simulink model "Wind_PMSG_Rectifier"  (Simulink 7.1)
settings: Solver=ode23tb  StartTime=0.0  StopTime=10.0  RelTol=1e-3
undefined symbols (not defined in the file or in its folder): c1, c2, c3, c4, c5, c6, DiscIntNeverNeededParam
libraries: powerlib x20, powerlib_extras x10, simulink x1
settings Model: Creator=jagan  LastModifiedBy=jagan

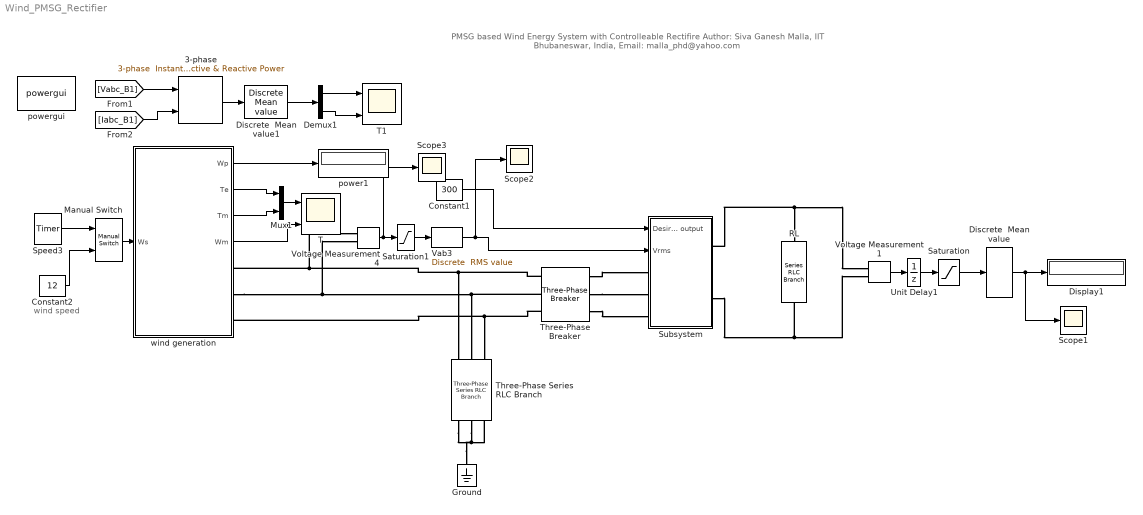
== system Wind_PMSG_Rectifier ==
  note: wind speed
  note: PMSG based Wind Energy System with Controlleable Rectifire
      | Author: Siva Ganesh Malla, IIT Bhubaneswar, India, Email: malla_phd@yahoo.com
  "3-phase " : powerlib_extras/Measurements/3-phase  Instantaneous  Active & Reactive Power  DialogController=POWERSYS.PowerSysDialog  SystemSampleTime=-1
  Constant1 : Constant  Value=300  OutDataType=sfix(16)  OutScaling=2^0
  Constant2 : Constant  Value=12  OutDataType=sfix(16)  OutScaling=2^0
  Demux1 : Demux  Outputs=2
  Discrete  Mean value : powerlib_extras/Discrete Measurements/Discrete  Mean value  DialogController=POWERSYS.PowerSysDialog  SystemSampleTime=-1  Freq=50*6  Vinit=0  Ts=50e-6
  Discrete  Mean value1 : powerlib_extras/Discrete Measurements/Discrete  Mean value  DialogController=POWERSYS.PowerSysDialog  SystemSampleTime=-1  Freq=50  Vinit=0  Ts=20e-6
  Display1 : Display
  Ground : powerlib/Elements/Ground  Orientation=down  DialogController=POWERSYS.PowerSysDialog  PhysicalDomain=powersysdomain  SubClassName=unknown  LeftPortType=p1  RightPortType=p1  LConnTagsString=a
  Manual Switch : simulink/Signal Routing/Manual Switch  SystemSampleTime=-1  sw=0  action=0  varsize=off
  Mux1 : Mux  Inputs=2
  RL : powerlib/Elements/Series RLC Branch  Orientation=down  DialogController=POWERSYS.PowerSysDialog  PhysicalDomain=powersysdomain  SubClassName=unknown  LeftPortType=p1  RightPortType=p1  LConnTagsString=__new0  RConnTagsString=__new0  BranchType=RL  Resistance=10  Inductance=50e-3  SetiL0=off  InitialCurrent=0  Capacitance=1e-6  Setx0=off  InitialVoltage=0  Measurements=None
  Saturation : Saturate  UpperLimit=1000  LowerLimit=-1000  OutDataType=sfix(16)  OutScaling=2^0
  Saturation1 : Saturate  UpperLimit=1000  LowerLimit=-1000  OutDataType=sfix(16)  OutScaling=2^0
  Scope1 : Scope
      settings: TimeRange=0.02  YMin=270  YMax=355  SaveName=ScopeData3
  Scope2 : Scope
      settings: TimeRange=0.02  YMin=423  YMax=438  SaveName=ScopeData5
  Scope3 : Scope
      settings: TimeRange=0.02  YMin=-1000  YMax=700  SaveName=ScopeData6
  Speed3 : powerlib_extras/Control  Blocks/Timer  DialogController=POWERSYS.PowerSysDialog  SystemSampleTime=-1  t=[0 3 5]  e=[12 7 12]
  Subsystem : Subsystem
  T : Scope  NumInputPorts=2
      settings: YMin=39.75~152.46  YMax=39.97~152.59  SaveName=Wind_MPPT  SampleInput=on  SampleTime=100e-6
  T1 : Scope  NumInputPorts=2
      settings: YMin=4380~-4e-014  YMax=4520~3.5e-014  SaveName=Wind_MPPT1  SampleInput=on  SampleTime=100e-6
  Three-Phase Series RLC Branch : powerlib/Elements/Three-Phase Series RLC Branch  Orientation=down  DialogController=POWERSYS.PowerSysDialog  PhysicalDomain=powersysdomain  SubClassName=unknown  LeftPortType=p1  RightPortType=p1  LConnTagsString=A|B|C  RConnTagsString=A|B|C  BranchType=R  Resistance=800  Inductance=1e-3  Capacitance=1e-6  Measurements=None
  Three-Phase Breaker : powerlib/Elements/Three-Phase Breaker  DialogController=POWERSYS.PowerSysDialog  SystemSampleTime=-1  InitialState=open  SwitchA=on  SwitchB=on  SwitchC=on  SwitchTimes=[1 10]  External=off  BreakerResistance=0.001  SnubberResistance=1e6  SnubberCapacitance=inf  Measurements=None
  Unit Delay1 : UnitDelay  SampleTime=-1
  Vab3 : powerlib_extras/Discrete Measurements/Discrete  RMS value  DialogController=POWERSYS.PowerSysDialog  SystemSampleTime=-1  Freq=50  Mag_Init=0  Ts=20e-6
  Voltage Measurement1 : powerlib/Measurements/Voltage Measurement  DialogController=POWERSYS.PowerSysDialog  SystemSampleTime=-1  PhasorSimulation=off  OutputType=Complex  PSBequivalent=0
  Voltage Measurement4 : powerlib/Measurements/Voltage Measurement  DialogController=POWERSYS.PowerSysDialog  SystemSampleTime=-1  PhasorSimulation=off  OutputType=Complex  PSBequivalent=0
  power1 : Display
      settings: SampleTime=1e-3
  powergui : powerlib/powergui  SystemSampleTime=-1  SimulationMode=Discrete  SampleTime=20e-6  frequency=60  SPID=off  SwTol=0  Interpol=off  x0status=blocks  echomessages=off  HookPort=off  FunctionMessages=off  EnableUseOfTLC=off  RestoreLinks=warning  frequencyindice=0  Frange=[0:2:500]  Ylog=off  Xlog=on  ShowGrid=off  save=off  variable=ZData  ZoomFFT=on  StartTime=0.0  cycles=1  DisplayStyle=1  fundamental=60  FreqAxis=off  MaxFrequency=1000  frequencyindicesteady=1  RmsSteady=1  display=off  Ts=0  methode=off
  wind generation : Subsystem
  wires:
  [Vabc_B1] -> "3-phase "/1
  [Iabc_B1] -> "3-phase "/2
  "3-phase "/1 -> Discrete  Mean value1/1
  Discrete  Mean value1/1 -> Demux1/1
  Demux1/1 -> T1/1
  Speed3/1 -> Manual Switch/1
  Constant2/1 -> Manual Switch/2
  Manual Switch/1 -> wind generation/1(Ws)
  Mux1/1 -> T/1
  wind generation/1(Wp) -> power1/1
  wind generation/2(Te) -> Mux1/1
  wind generation/3(Tm) -> Mux1/2
  wind generation/4(Wm) -> T/2
  Demux1/2 -> T1/2
  Voltage Measurement4/1 -> Saturation1/1, Scope3/1
  Saturation1/1 -> Vab3/1
  Vab3/1 -> Subsystem/2(Vrms), Scope2/1
  Constant1/1 -> Subsystem/1(Desird output)
  Discrete  Mean value/1 -> Display1/1, Scope1/1
  Voltage Measurement1/1 -> Unit Delay1/1
  Saturation/1 -> Discrete  Mean value/1
  Unit Delay1/1 -> Saturation/1
  connections:
  wind generation/RConn2 -- Voltage Measurement4/LConn2 -- Three-Phase Breaker/LConn2 -- Three-Phase Series RLC Branch/LConn2
  Three-Phase Breaker/RConn1 -- Subsystem/LConn1
  Three-Phase Breaker/RConn3 -- Subsystem/LConn3
  Subsystem/RConn1 -- Voltage Measurement1/LConn1 -- RL/LConn1
  Subsystem/RConn2 -- Voltage Measurement1/LConn2 -- RL/RConn1
  wind generation/RConn3 -- Three-Phase Breaker/LConn3 -- Three-Phase Series RLC Branch/LConn3
  Three-Phase Breaker/RConn2 -- Subsystem/LConn2
  Three-Phase Breaker/LConn1 -- Three-Phase Series RLC Branch/LConn1 -- wind generation/RConn1 -- Voltage Measurement4/LConn1
  Ground/LConn1 -- Three-Phase Series RLC Branch/RConn1 -- Three-Phase Series RLC Branch/RConn3 -- Three-Phase Series RLC Branch/RConn2

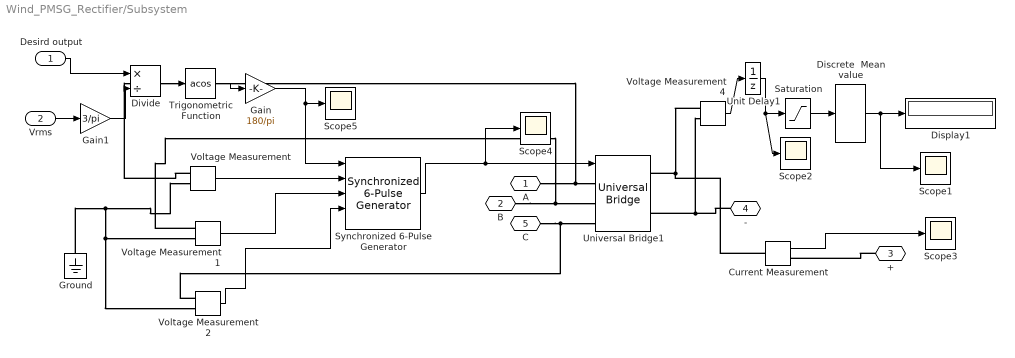
== system Wind_PMSG_Rectifier/Subsystem ==
  Desird output : Inport
  Vrms : Inport  Port=2
  Current Measurement : powerlib/Measurements/Current Measurement  DialogController=POWERSYS.PowerSysDialog  SystemSampleTime=-1  PhasorSimulation=off  OutputType=Complex  PSBequivalent=0
  Discrete  Mean value : powerlib_extras/Discrete Measurements/Discrete  Mean value  DialogController=POWERSYS.PowerSysDialog  SystemSampleTime=-1  Freq=50*6  Vinit=0  Ts=50e-6
  Display1 : Display
  Divide : Product  Inputs=*/  OutDataType=sfix(16)  OutScaling=2^-10
  Gain : Gain  Gain=180/pi  ParameterDataType=sfix(16)  ParameterScaling=2^0  OutDataType=sfix(16)  OutScaling=2^0
  Gain1 : Gain  Gain=3/pi  ParameterDataType=sfix(16)  ParameterScaling=2^0  OutDataType=sfix(16)  OutScaling=2^0
  Ground : powerlib/Elements/Ground  Orientation=down  DialogController=POWERSYS.PowerSysDialog  PhysicalDomain=powersysdomain  SubClassName=unknown  LeftPortType=p1  RightPortType=p1  LConnTagsString=a
  Saturation : Saturate  UpperLimit=1000  LowerLimit=-1000  OutDataType=sfix(16)  OutScaling=2^0
  Scope{1..5} (5 alike) : Scope
      Scope1 settings: TimeRange=0.02  YMin=-25  YMax=325
      Scope2 settings: TimeRange=0.02  YMin=-250  YMax=550
      Scope3 settings: TimeRange=0.02  YMin=25.75  YMax=28.5  SaveName=ScopeData2
      Scope4 settings: TimeRange=0.02  YMin=0  YMax=1  SaveName=ScopeData4
      Scope5 settings: TimeRange=0.02  YMin=-1  YMax=1  SaveName=ScopeData7
  Synchronized 6-Pulse Generator : powerlib_extras/Control  Blocks/Synchronized 6-Pulse Generator  DialogController=POWERSYS.PowerSysDialog  SystemSampleTime=-1  freq=25  pwidth=50  Double_Pulse=off
  Trigonometric Function : Trigonometry  Operator=acos
  Unit Delay1 : UnitDelay  SampleTime=-1
  Universal Bridge1 : powerlib/Power Electronics/Universal Bridge  DialogController=POWERSYS.PowerSysDialog  SystemSampleTime=-1  Arms=3  SnubberResistance=1e5  SnubberCapacitance=inf  Device=Thyristors  Ron=1e-3  Lon=0  ForwardVoltages="[  0  0  ]"  ForwardVoltage=0  GTOparameters=[ 10e-6 , 20e-6 ]  IGBTparameters=[ 1e-6 , 2e-6 ]  Measurements=None  converterType=Rectifier
  Voltage Measurement{,1..2,4} (4 alike) : powerlib/Measurements/Voltage Measurement  DialogController=POWERSYS.PowerSysDialog  SystemSampleTime=-1  PhasorSimulation=off  OutputType=Complex  PSBequivalent=0
  A : PMIOPort  Port=1  Side=Left
  B : PMIOPort  Port=2  Side=Left
  + : PMIOPort  Orientation=left  Port=3  Side=Right
  - : PMIOPort  Orientation=left  Port=4  Side=Right
  C : PMIOPort  Port=5  Side=Left
  wires:
  Voltage Measurement/1 -> Synchronized 6-Pulse Generator/2
  Voltage Measurement1/1 -> Synchronized 6-Pulse Generator/3
  Voltage Measurement2/1 -> Synchronized 6-Pulse Generator/4
  Synchronized 6-Pulse Generator/1 -> Universal Bridge1/1, Scope4/1
  Voltage Measurement4/1 -> Unit Delay1/1
  Current Measurement/1 -> Scope3/1
  Divide/1 -> Trigonometric Function/1
  Trigonometric Function/1 -> Gain/1
  Gain/1 -> Synchronized 6-Pulse Generator/1, Scope5/1
  Discrete  Mean value/1 -> Display1/1, Scope1/1
  Desird output/1 -> Divide/1
  ? -> Synchronized 6-Pulse Generator/5
  Gain1/1 -> Divide/2
  Vrms/1 -> Gain1/1
  Saturation/1 -> Discrete  Mean value/1
  Unit Delay1/1 -> Scope2/1, Saturation/1
  connections:
  Current Measurement/LConn1 -- Voltage Measurement4/LConn1 -- Universal Bridge1/RConn1
  A/RConn1 -- Universal Bridge1/LConn1 -- Voltage Measurement/LConn1
  -/RConn1 -- Universal Bridge1/RConn2 -- Voltage Measurement4/LConn2
  Voltage Measurement2/LConn1 -- C/RConn1 -- Universal Bridge1/LConn3
  +/RConn1 -- Current Measurement/RConn1
  Voltage Measurement1/LConn1 -- B/RConn1 -- Universal Bridge1/LConn2
  Voltage Measurement/LConn2 -- Ground/LConn1 -- Voltage Measurement2/LConn2 -- Voltage Measurement1/LConn2

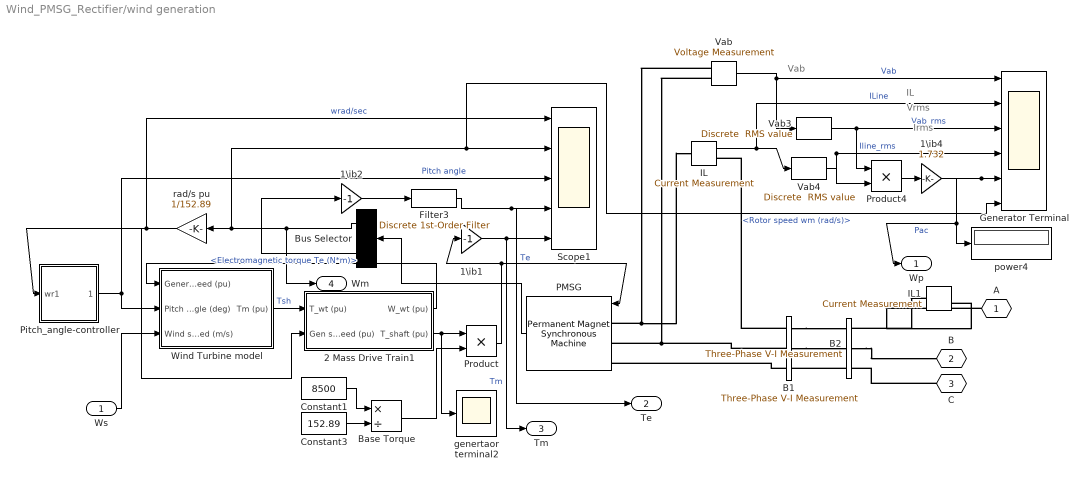
== system Wind_PMSG_Rectifier/wind generation ==
  note: Vab
  note: IL
  note: Vrms
  note: Irms
  Ws : Inport  OutDataType=sfix(16)  OutScaling=2^0
  1\ib1 : Gain  Gain=-1  ParameterDataType=sfix(16)  ParameterScaling=2^0  OutDataType=sfix(16)  OutScaling=2^0  SaturateOnIntegerOverflow=on  OutDataTypeStr=Inherit: Same as input  ParamDataTypeStr=Inherit: Same as input
  1\ib2 : Gain  Gain=-1  ParameterDataType=sfix(16)  ParameterScaling=2^0  OutDataType=sfix(16)  OutScaling=2^0  SaturateOnIntegerOverflow=on  OutDataTypeStr=Inherit: Same as input  ParamDataTypeStr=Inherit: Same as input
  1\ib4 : Gain  Gain=1.732  ParameterDataType=sfix(16)  ParameterScaling=2^0  OutDataType=sfix(16)  OutScaling=2^0  SaturateOnIntegerOverflow=on  OutDataTypeStr=Inherit: Same as input  ParamDataTypeStr=Inherit: Same as input
  2 Mass Drive Train1 : Subsystem
  B1 : powerlib/Measurements/Three-Phase V-I Measurement  DialogController=POWERSYS.PowerSysDialog  SystemSampleTime=-1  VoltageMeasurement=phase-to-ground  SetLabelV=on  LabelV=Vabc_B1  Vpu=off  CurrentMeasurement=yes  SetLabelI=on  LabelI=Iabc_B1  Ipu=off  Pbase=100e6  Vbase=500e3  OutputType=Magnitude  PhasorSimulation=off  PSBequivalent=0
  "B2 " : powerlib/Measurements/Three-Phase V-I Measurement  DialogController=POWERSYS.PowerSysDialog  SystemSampleTime=-1  VoltageMeasurement=no  SetLabelV=on  LabelV=Vabc_B2  Vpu=off  CurrentMeasurement=no  SetLabelI=on  LabelI=Iabc_B2  Ipu=off  Pbase=100e6  Vbase=500e3  OutputType=Magnitude  PhasorSimulation=off  PSBequivalent=0
  Base Torque : Product  Inputs=*/  OutDataType=sfix(16)  OutScaling=2^0  RndMeth=Zero
  Bus Selector : BusSelector  Orientation=left  OutputSignals=Rotor speed wm (rad/s),Electromagnetic torque Te (N*m)
  Constant1 : Constant  Value=8500  OutDataType=sfix(16)  OutScaling=2^0
  Constant3 : Constant  Value=152.89  OutDataType=sfix(16)  OutScaling=2^0
  Filter3 : powerlib_extras/Discrete  Control Blocks/Discrete 1st-Order Filter  DialogController=POWERSYS.PowerSysDialog  SystemSampleTime=-1  FilterType=Lowpass  Tc=1e-3  Ts=20e-6  Initialize=off  Vac_Init=[0.8 -25 60]  Vdc_Init=-0.4  PlotResponse=off  param1=[1 500 0.1]
  Generator Terminal : Scope  NumInputPorts=6
      settings: YMin=-750~-1~450~0.525~410~175.15  YMax=750~1~477.5~0.56~460~175.4  SaveName=Generator_Terminal  SampleInput=on  SampleTime=100e-6
  IL : powerlib/Measurements/Current Measurement  DialogController=POWERSYS.PowerSysDialog  SystemSampleTime=-1  PhasorSimulation=off  OutputType=Complex  PSBequivalent=0
  IL1 : powerlib/Measurements/Current Measurement  DialogController=POWERSYS.PowerSysDialog  SystemSampleTime=-1  PhasorSimulation=off  OutputType=Complex  PSBequivalent=0
  PMSG : powerlib/Machines/Permanent Magnet Synchronous Machine  Orientation=left  DialogController=POWERSYS.PowerSysDialog  SystemSampleTime=-1  FluxDistribution=Sinusoidal  MechanicalLoad=Torque Tm  PresetModel=No  ShowDetailedParameters=on  Resistance=0.425  Inductance=8.5e-3  dqInductances=[0.0082 0.0082]  MachineConstant=Flux linkage established by magnets (V.s)  Flux=0.433  VoltageCst=392.6876  TorqueCst=3.2475  Flat=120  Mechanical=[0.01197 0.001189 5]  PolePairs=5  InitialConditions=[0,0, 0,0]  TsPowergui=0  TsBlock=-1
  Pitch_angle-controller : Subsystem
  Product : Product  OutDataType=sfix(16)  OutScaling=2^0  RndMeth=Zero
  Product4 : Product  OutDataType=sfix(16)  OutScaling=2^0  RndMeth=Zero
  Scope1 : Scope  NumInputPorts=5
      settings: YMin=0.993~151.8~-1~37.5~40.05  YMax=1~152.8~1~42.5~40.325  SaveName=ScopeData90  SampleInput=on  SampleTime=100e-6
  Vab : powerlib/Measurements/Voltage Measurement  DialogController=POWERSYS.PowerSysDialog  SystemSampleTime=-1  PhasorSimulation=off  OutputType=Complex  PSBequivalent=0
  Vab3 : powerlib_extras/Discrete Measurements/Discrete  RMS value  DialogController=POWERSYS.PowerSysDialog  SystemSampleTime=-1  Freq=50  Mag_Init=0  Ts=20e-6
  Vab4 : powerlib_extras/Discrete Measurements/Discrete  RMS value  DialogController=POWERSYS.PowerSysDialog  SystemSampleTime=-1  Freq=50  Mag_Init=0  Ts=20e-6
  Wind Turbine model : Subsystem  AncestorBlock=DRlib/Wind Generation/Wind Turbine  DialogController=POWERSYS.PowerSysDialog  mask(Wind Turbine){Pnom=8.5e3, Pelec_base=8.5e3/0.9, wind_base=12, P_wind_base=0.8, speed_nom=1, pitch_angle=0, DisplayTurbChar=off, c1_c6=[0.51763          116          0.4            5           21     0.006795], cp_nom=0.48, lambda_nom=8.1}
      mask prompts: Pnom "Nominal mechanical output power (W):"; Pelec_base "Base power of the electrical generator (VA):"; wind_base "Base wind speed (m/s):"; P_wind_base "Maximum power at base wind speed (pu of nominal mechanical power):"; speed_nom "Base rotational speed (p.u. of base generator speed):"; pitch_angle "Pitch angle beta to display wind-turbine power characteristics (beta >=0)  (deg):"; DisplayTurbChar "Display wind turbine power characteristics"
      mask help:
      | This block implements a variable pitch wind turbine model. The performance coefficient Cp of the turbine is the mechanical output power of the turbine divided by wind power and a function of wind speed, rotational speed, and pitch angle (beta). Cp reaches its maximum value at zero beta. Select the wind-turbine power characteristics display to plot the turbine characteristics at the specified pitch angle.
      |
      | The first input is the generator speed in per unit of the generator base speed. For a synchronous or asynchronous generator, the base speed is the synchronous speed. For a permanent-magnet generator, the base speed is defined as the speed producing nominal voltage at  no load. The second input is the blade pitch angle (beta) in degrees. The third input is the wind speed in m/s.
      |
      | The output is the torque applied to the generator shaft in per unit of the generator ratings.
      |
      | The turbine inertia must be added to the generator inertia.
      mask init:
      | %Wind turbine typical characteristic data
      | %c2=116;c3=0.4;c4=5;c5=21;
      | %Computation of c1 and c6 for lambda_nom et cpmax
      | %lambda_nom=8.1;
      | %cp_max=0.48;
      | %cp_nom=cp_max;
      | 
      | %lambda_i_nom=1/(1/lambda_nom-0.035);
      | %k_nom=-(c2*c5/lambda_i_nom-c4*c5-c2)*exp(-c5/lambda_i_nom)/lambda_nom^2;
      | %c1=cp_max/((c2/lambda_i_nom-c4)*exp(-c5/lambda_i_nom)+k_nom*lambda_nom);
      | %c6=k_nom*c1;
      | power_initmask();
      mask Help: web(psbhelp);
      mask CallbackString:
      | ParVisible={'on','on','on','on','on','on','on','off','off','off',};
      | set_param(gcb,'MaskVisibilities',ParVisible);
      | c1_c6=str2num(get_param(gcb,'c1_c6'));
      | c1=c1_c6(1);c2=c1_c6(2);c3=c1_c6(3);c4=c1_c6(4);c5=c1_c6(5);c6=c1_c6(6);||||||DisplayTurbChar=get_param(gcb,'DisplayTurbChar');
      | 
      | if strcmp(DisplayTurbChar,'on')
      |     fig_num=figure;
      | 	clf(fig_num);
      | 	[speed_nom,wind_base,P_wind_base,pitch_angle]=getSPSmaskvalues(gcb,{'speed_nom','wind_base','P_wind_base','pitch_angle'});
      | 	[c1_c6,lambda_nom,cp_nom]=getSPSmaskvalues(gcb,{'c1_c6','lambda_nom','cp_nom'});
      | 	c1=c1_c6(1);c2=c1_c6(2);c3=c1_c6(3);c4=c1_c6(4);c5=c1_c6(5);c6=c1_c6(6);
      | 
      | 	%Wind turbine typical characteristic data
      |     %c2=116;c3=0.4;c4=5;c5=21;
      |     %Computation of c1 and c6 for lambda_nom et cpmax
      |     %lambda_nom=8.1;
      |     %cp_max=0.48;
      |     %cp_nom=cp_max;
      | 
      |     %lambda_i_nom=1/(1/lambda_nom-0.035);
      |     %k_nom=-(c2*c5/lambda_i_nom-c4*c5-c2)*exp(-c5/lambda_i_nom)/lambda_nom^2;
      |     %c1=cp_max/((c2/lambda_i_nom-c4)*exp(-c5/lambda_i_nom)+k_nom*lambda_nom);
      |     %c6=k_nom*c1;
      | 
      | 	wr_elec_pu=1e-3:0.01:1.5;;
      |     wr_mec_pu=wr_elec_pu/speed_nom;
      |     wind_max=ceil((1.2/P_wind_base)^(1/3)*wind_base);
      |     wind_min=round(((0.1)/P_wind_base)^(1/3)*wind_base);
      |     wind1=wind_min:(wind_base-wind_min)/5:wind_base;
      |     wind2=wind_base+(wind_base-wind_min)/5:(wind_base-wind_min)/5:wind_max;
      |     wind_pu=[wind1 wind2]/wind_base;
      | 
      |     for k=1:length(wind_pu)
      |         for i=1:length(wr_mec_pu);
      |             lambda_pu=wr_mec_pu(i)/wind_pu(k);
      |             lambda=lambda_pu*lambda_nom;
      |             lambda_i=1/(1/(lambda+0.08*pitch_angle)-0.035/(pitch_angle^3+1));
      |             cp=c1*(c2/lambda_i-c3*pitch_angle-c4)*exp(-c5/lambda_i)+c6*lambda;
      |             cp_pu=cp/cp_nom;
      |             Pwind_pu(k,i)=wind_pu(k)^3*cp_pu*P_wind_base;
      |         end
      |     end
      |     for k=1:length(wind_pu)
      |         plot(wr_elec_pu,Pwind_pu(k,:))
      |         hold on
      |     end
      | 
      |     plot([speed_nom,speed_nom,0],[0,P_wind_base,P_wind_base],'r--')
      |     text(speed_nom+0.01,0+0.05,sprintf('%0.4g pu',speed_nom))
      |     text(0.01,P_wind_base+0.05,sprintf('Max. power at base wind speed (%0.4g m/s) and beta = 0 deg',wind_base))
      |     for i=1:length(wind_pu),
      |         p_max(i)=max(Pwind_pu(i,:));
      |         speed(i)=wr_elec_pu(find(Pwind_pu(i,:)==p_max(i)));
      |         text(speed(i),p_max(i),sprintf('%0.4g m/s',wind_pu(i)*wind_base))
      |     end
      |     plot([0 max(wr_elec_pu)],[0 0],'--')
      | 
      |     xlabel('Turbine speed (pu of nominal generator speed)')
      |     ylabel('Turbine output power (pu of nominal mechanical power)')
      |     title(sprintf('Turbine Power Characteristics (Pitch angle beta = %0.4g deg)',pitch_angle))
      |     axis([0 max(wr_elec_pu) min(Pwind_pu(1,:)) max(P_wind_base+0.1,max(wind_pu)^3*P_wind_base+0.1)])
      |     set_param(gcb,'DisplayTurbChar','off')
      | end|||
      mask Display: disp('');
  genertaor terminal2 : Scope
      settings: YMin=-0.5138  YMax=-0.5122  SaveName=ref_torque1  SampleInput=on  SampleTime=100e-6
  power4 : Display
      settings: SampleTime=1e-3
  rad/s pu : Gain  Orientation=left  Gain=1/152.89  ParameterDataType=sfix(16)  ParameterScaling=2^0  OutDataType=sfix(16)  OutScaling=2^0  SaturateOnIntegerOverflow=on  OutDataTypeStr=Inherit: Same as input  ParamDataTypeStr=Inherit: Same as input
  A : PMIOPort  Tag=PMCPort  Orientation=left  Port=1  Side=Right
  B : PMIOPort  Tag=PMCPort  Orientation=left  Port=2  Side=Right
  C : PMIOPort  Tag=PMCPort  Orientation=left  Port=3  Side=Right
  Wp : Outport  OutDataType=sfix(16)  OutScaling=2^0
  Te : Outport  Port=2  OutDataType=sfix(16)  OutScaling=2^0
  Tm : Outport  Port=3  OutDataType=sfix(16)  OutScaling=2^0
  Wm : Outport  Port=4  OutDataType=sfix(16)  OutScaling=2^0
  wires:
  Bus Selector/1 -> rad/s pu/1, Scope1/2, Generator Terminal/6, Wm/1  "<Rotor speed wm (rad/s)>"
  rad/s pu/1 -> Scope1/1, Pitch_angle-controller/1(wr1), 2 Mass Drive Train1/2(Gen speed (pu))  "wrad/sec"
  Vab/1 -> Vab3/1, Generator Terminal/1  "Vab"
  IL/1 -> Vab4/1, Generator Terminal/2  "ILine"
  Product4/1 -> 1\ib4/1
  1\ib1/1 -> Scope1/5, Tm/1  "Tm"
  1\ib2/1 -> Filter3/1
  Vab3/1 -> Product4/1, Generator Terminal/3  "Vab_rms"
  Vab4/1 -> Product4/2, Generator Terminal/4  "Iline_rms"
  1\ib4/1 -> Generator Terminal/5, power4/1, Wp/1  "Pac"
  Filter3/1 -> Scope1/4, Te/1  "Te"
  Product/1 -> PMSG/1, 1\ib1/1
  Pitch_angle-controller/1(Pitch_angle1) -> Scope1/3, Wind Turbine model/2(Pitch angle (deg))  "Pitch angle"
  Constant1/1 -> Base Torque/1
  Constant3/1 -> Base Torque/2
  PMSG/1 -> Bus Selector/1
  Bus Selector/2 -> 1\ib2/1  "<Electromagnetic torque Te (N*m)>"
  Ws/1 -> Wind Turbine model/3(Wind speed (m/s))
  Wind Turbine model/1(Tm (pu)) -> 2 Mass Drive Train1/1(T_wt (pu))  "Tsh"
  Base Torque/1 -> Product/2
  2 Mass Drive Train1/1(W_wt (pu)) -> Wind Turbine model/1(Generator speed (pu))
  2 Mass Drive Train1/2(T_shaft (pu)) -> Product/1, genertaor terminal2/1
  connections:
  B1/LConn1 -- IL/RConn1
  B1/LConn2 -- PMSG/LConn2 -- Vab/LConn2
  B1/LConn3 -- PMSG/LConn3
  B1/RConn1 -- "B2 "/LConn1
  B1/RConn2 -- "B2 "/LConn2
  "B2 "/LConn3 -- B1/RConn3
  IL1/LConn1 -- "B2 "/RConn1
  "B2 "/RConn2 -- B/RConn1
  C/RConn1 -- "B2 "/RConn3
  IL/LConn1 -- Vab/LConn1 -- PMSG/LConn1
  A/RConn1 -- IL1/RConn1

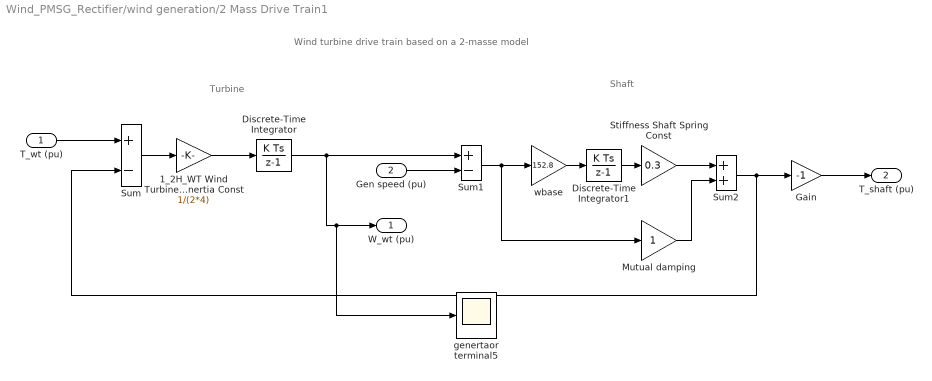
== system Wind_PMSG_Rectifier/wind generation/2 Mass Drive Train1 ==
  note: Wind turbine drive train based on a 2-masse model
  note: Turbine
  note: Shaft
  T_wt (pu) : Inport  OutDataType=sfix(16)  OutScaling=2^0
  Gen speed (pu) : Inport  Port=2  OutDataType=sfix(16)  OutScaling=2^0
  1_2H_WT Wind Turbine Inertia Const : Gain  Gain=1/(2*4)  ParameterDataType=sfix(16)  ParameterScaling=2^0  OutDataType=sfix(16)  OutScaling=2^0  SaturateOnIntegerOverflow=on  OutDataTypeStr=Inherit: Same as input  ParamDataTypeStr=Inherit: Same as input
  Discrete-Time Integrator : DiscreteIntegrator  InitialCondition=1  SampleTime=20e-6  OutDataType=sfix(16)  OutScaling=2^0  ICPrevOutput=DiscIntNeverNeededParam  ICPrevScaledInput=DiscIntNeverNeededParam
  Discrete-Time Integrator1 : DiscreteIntegrator  InitialCondition=1/0.3  SampleTime=20e-6  OutDataType=sfix(16)  OutScaling=2^0  UpperSaturationLimit=4  LowerSaturationLimit=-4  ICPrevOutput=DiscIntNeverNeededParam  ICPrevScaledInput=DiscIntNeverNeededParam
  Gain : Gain  Gain=-1  ParameterDataType=sfix(16)  ParameterScaling=2^0  OutDataType=sfix(16)  OutScaling=2^0  SaturateOnIntegerOverflow=on  OutDataTypeStr=Inherit: Same as input  ParamDataTypeStr=Inherit: Same as input
  Mutual damping : Gain  ParameterDataType=sfix(16)  ParameterScaling=2^0  OutDataType=sfix(16)  OutScaling=2^0  SaturateOnIntegerOverflow=on  OutDataTypeStr=Inherit: Same as input  ParamDataTypeStr=Inherit: Same as input
  Stiffness Shaft Spring Const : Gain  Gain=0.3  ParameterDataType=sfix(16)  ParameterScaling=2^0  OutDataType=sfix(16)  OutScaling=2^0  SaturateOnIntegerOverflow=on  OutDataTypeStr=Inherit: Same as input  ParamDataTypeStr=Inherit: Same as input
  Sum : Sum  Inputs=+-  OutDataType=sfix(16)  OutScaling=2^0  SaturateOnIntegerOverflow=on  InputSameDT=on  OutDataTypeStr=Inherit: Same as first input
  Sum1 : Sum  Inputs=+-  OutDataType=sfix(16)  OutScaling=2^0  SaturateOnIntegerOverflow=on  InputSameDT=on  OutDataTypeStr=Inherit: Same as first input
  Sum2 : Sum  OutDataType=sfix(16)  OutScaling=2^0  SaturateOnIntegerOverflow=on  InputSameDT=on  OutDataTypeStr=Inherit: Same as first input
  genertaor terminal5 : Scope
      settings: YMin=0.94175  YMax=0.94425  SaveName=Wwt  SampleInput=on  SampleTime=100e-6
  wbase : Gain  Gain=152.8  ParameterDataType=sfix(16)  ParameterScaling=2^0  OutDataType=sfix(16)  OutScaling=2^0  SaturateOnIntegerOverflow=on  OutDataTypeStr=Inherit: Same as input  ParamDataTypeStr=Inherit: Same as input
  W_wt (pu) : Outport  OutDataType=sfix(16)  OutScaling=2^0
  T_shaft (pu) : Outport  Port=2  OutDataType=sfix(16)  OutScaling=2^0
  wires:
  T_wt (pu)/1 -> Sum/1
  Sum2/1 -> Sum/2, Gain/1
  Mutual damping/1 -> Sum2/2
  Sum1/1 -> Mutual damping/1, wbase/1
  Gen speed (pu)/1 -> Sum1/2
  Discrete-Time Integrator/1 -> Sum1/1, W_wt (pu)/1, genertaor terminal5/1
  1_2H_WT Wind Turbine Inertia Const/1 -> Discrete-Time Integrator/1
  Sum/1 -> 1_2H_WT Wind Turbine Inertia Const/1
  Stiffness Shaft Spring Const/1 -> Sum2/1
  Discrete-Time Integrator1/1 -> Stiffness Shaft Spring Const/1
  wbase/1 -> Discrete-Time Integrator1/1
  Gain/1 -> T_shaft (pu)/1

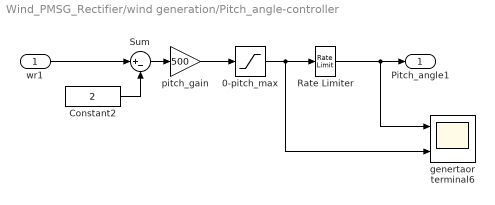
== system Wind_PMSG_Rectifier/wind generation/Pitch_angle-controller ==
  wr1 : Inport  OutDataType=sfix(16)  OutScaling=2^0
  0-pitch_max : Saturate  UpperLimit=45  LowerLimit=0
  Constant2 : Constant  Value=2  OutDataType=sfix(16)  OutScaling=2^0
  "Rate Limiter   " : RateLimiter  RisingSlewLimit=2  FallingSlewLimit=-2
  Sum : Sum  Inputs=|+-  OutDataType=sfix(16)  OutScaling=2^0  SaturateOnIntegerOverflow=on
  genertaor terminal6 : Scope  NumInputPorts=2
      settings: YMin=-1~-1  YMax=1~1  SaveName=ScopeData9  SampleInput=on  SampleTime=100e-6
  pitch_gain : Gain  Gain=500  ParameterDataType=sfix(16)  ParameterScaling=2^0  OutDataType=sfix(16)  OutScaling=2^0  SaturateOnIntegerOverflow=on  OutDataTypeStr=Inherit: Same as input  ParamDataTypeStr=Inherit: Same as input
  Pitch_angle1 : Outport  OutDataType=sfix(16)  OutScaling=2^0
  wires:
  "Rate Limiter   "/1 -> Pitch_angle1/1, genertaor terminal6/1
  pitch_gain/1 -> 0-pitch_max/1
  Sum/1 -> pitch_gain/1
  Constant2/1 -> Sum/2
  0-pitch_max/1 -> "Rate Limiter   "/1, genertaor terminal6/2
  wr1/1 -> Sum/1

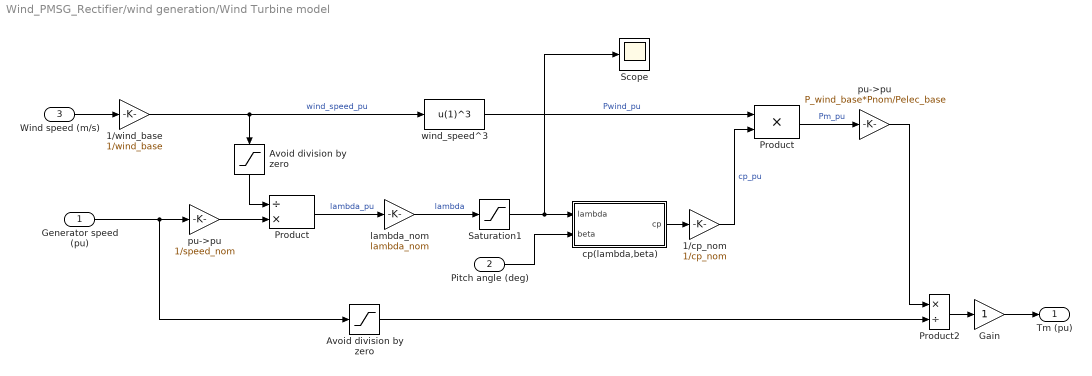
== system Wind_PMSG_Rectifier/wind generation/Wind Turbine model ==
  Generator speed (pu) : Inport  OutDataType=sfix(16)  OutScaling=2^0
  Pitch angle (deg) : Inport  Port=2  OutDataType=sfix(16)  OutScaling=2^0
  Wind speed (m/s) : Inport  Port=3  OutDataType=sfix(16)  OutScaling=2^0
  1/cp_nom : Gain  Gain=1/cp_nom  ParameterDataType=sfix(16)  ParameterScaling=2^0  OutDataType=sfix(16)  OutScaling=2^0  SaturateOnIntegerOverflow=on  OutDataTypeStr=Inherit: Same as input  ParamDataTypeStr=Inherit: Same as input
  1/wind_base : Gain  Gain=1/wind_base  ParameterDataType=sfix(16)  ParameterScaling=2^0  OutDataType=sfix(16)  OutScaling=2^0  SaturateOnIntegerOverflow=on  OutDataTypeStr=Inherit: Same as input  ParamDataTypeStr=Inherit: Same as input
  Avoid division by zero : Saturate  UpperLimit=1e6  LowerLimit=1e-6  OutDataType=sfix(16)  OutScaling=2^0
  "Avoid division by zero " : Saturate  Orientation=down  UpperLimit=1e6  LowerLimit=1e-6  OutDataType=sfix(16)  OutScaling=2^0
  Gain : Gain  ParameterDataType=sfix(16)  ParameterScaling=2^0  OutDataType=sfix(16)  OutScaling=2^0  SaturateOnIntegerOverflow=on  OutDataTypeStr=Inherit: Same as input  ParamDataTypeStr=Inherit: Same as input
  Product : Product  Inputs=/*  OutDataType=sfix(16)  OutScaling=2^0  SaturateOnIntegerOverflow=on  OutDataTypeStr=Inherit: Same as first input
  "Product " : Product  OutDataType=sfix(16)  OutScaling=2^0  SaturateOnIntegerOverflow=on  OutDataTypeStr=Inherit: Same as first input
  Product2 : Product  Inputs=*/  OutDataType=sfix(16)  OutScaling=2^0  SaturateOnIntegerOverflow=on  InputSameDT=on  OutDataTypeStr=Inherit: Same as first input
  Saturation1 : Saturate  UpperLimit=inf  LowerLimit=1e-6  OutDataType=sfix(16)  OutScaling=2^0
  Scope : Scope
      settings: SaveName=ScopeData10
  cp(lambda,beta) : Subsystem
  lambda_nom : Gain  Gain=lambda_nom  ParameterDataType=sfix(16)  ParameterScaling=2^0  OutDataType=sfix(16)  OutScaling=2^0  SaturateOnIntegerOverflow=on  OutDataTypeStr=Inherit: Same as input  ParamDataTypeStr=Inherit: Same as input
  pu->pu : Gain  Gain=P_wind_base*Pnom/Pelec_base  ParameterDataType=sfix(16)  ParameterScaling=2^0  OutDataType=sfix(16)  OutScaling=2^0  SaturateOnIntegerOverflow=on  OutDataTypeStr=Inherit: Same as input  ParamDataTypeStr=Inherit: Same as input
  "pu->pu " : Gain  Gain=1/speed_nom  ParameterDataType=sfix(16)  ParameterScaling=2^0  OutDataType=sfix(16)  OutScaling=2^0  SaturateOnIntegerOverflow=on  OutDataTypeStr=Inherit: Same as input  ParamDataTypeStr=Inherit: Same as input
  wind_speed^3 : Fcn  Expr=u(1)^3
  Tm (pu) : Outport  OutDataType=sfix(16)  OutScaling=2^0
  wires:
  Pitch angle (deg)/1 -> cp(lambda,beta)/2(beta)
  pu->pu/1 -> Product2/1
  cp(lambda,beta)/1(cp) -> 1/cp_nom/1
  wind_speed^3/1 -> "Product "/1  "Pwind_pu"
  Product2/1 -> Gain/1
  Avoid division by zero/1 -> Product2/2
  Wind speed (m/s)/1 -> 1/wind_base/1
  Gain/1 -> Tm (pu)/1
  Generator speed (pu)/1 -> Avoid division by zero/1, "pu->pu "/1
  "Product "/1 -> pu->pu/1  "Pm_pu"
  lambda_nom/1 -> Saturation1/1  "lambda"
  1/cp_nom/1 -> "Product "/2  "cp_pu"
  Saturation1/1 -> cp(lambda,beta)/1(lambda), Scope/1
  Product/1 -> lambda_nom/1  "lambda_pu"
  1/wind_base/1 -> wind_speed^3/1, "Avoid division by zero "/1  "wind_speed_pu"
  "Avoid division by zero "/1 -> Product/1
  "pu->pu "/1 -> Product/2

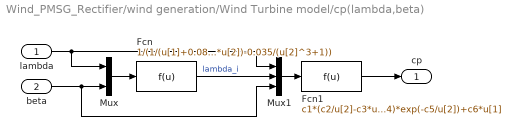
== system Wind_PMSG_Rectifier/wind generation/Wind Turbine model/cp(lambda,beta) ==
  lambda : Inport  OutDataType=sfix(16)  OutScaling=2^0
  beta : Inport  Port=2  OutDataType=sfix(16)  OutScaling=2^0
  Fcn : Fcn  Expr=1/(1/(u[1]+0.08*u[2])-0.035/(u[2]^3+1))
  Fcn1 : Fcn  Expr=c1*(c2/u[2]-c3*u[3]-c4)*exp(-c5/u[2])+c6*u[1]
  Mux : Mux  Inputs=2
  Mux1 : Mux  Inputs=3
  cp : Outport  OutDataType=sfix(16)  OutScaling=2^0
  wires:
  Fcn/1 -> Mux1/2  "lambda_i"
  Fcn1/1 -> cp/1
  lambda/1 -> Mux1/1, Mux/1
  Mux1/1 -> Fcn1/1
  beta/1 -> Mux1/3, Mux/2
  Mux/1 -> Fcn/1
